simulink model "gm_iir_filter_simulink"  (R2025a)
settings: Solver=FixedStepAuto  StartTime=0.0  StopTime=5e-3  MaxStep=1/(44e3)  RelTol=1e-3  EnableMultiTasking=on
libraries: hdlmdlgenlib x17
settings Model: Creator=thiag  LastModifiedBy=thiag
settings SolverCC: PositivePriorityOrder=on
settings OptimizationCC: BlockReduction=off  ConditionallyExecuteInputs=off  DefaultParameterBehavior=Inlined  EnhancedBackFolding=on  PassReuseOutputArgsAs=Individual arguments  ZeroExternalMemoryAtStartup=off  ZeroInternalMemoryAtStartup=off  MaxStackSize=64  OptimizeBlockOrder=speed  DifferentSizesBufferReuse=on  OptimizationCustomize=off  EfficientTunableParamExpr=on
settings DebuggingCC: InheritedTsInSrcMsg=none  ParameterTunabilityLossMsg=error
settings HardwareCC: ProdBitPerPointer=32.0  ProdBitPerSizeT=32.0  ProdBitPerPtrDiffT=32.0  ProdLargestAtomicInteger=Long  ProdLargestAtomicFloat=Double  ProdWordSize=32.0  ProdLongLongMode=on  ProdHWDeviceType=ARM Compatible->ARM Cortex-A (32-bit)  TargetBitPerPointer=64.0  TargetBitPerSizeT=64.0  TargetBitPerPtrDiffT=64.0  TargetLongLongMode=on  TargetIntDivRoundTo=Zero  TargetEndianess=LittleEndian  TargetWordSize=64.0  TargetHWDeviceType=Custom Processor->MATLAB Host Computer  ProdEqTarget=off
settings RTWCC: SystemTargetFile=ert.tlc  HardwareBoard=Altera Cyclone V SoC development kit  TLCOptions="-aInlineSetEventsForThisBaseRateFcn=TLC_FALSE -aSuppressMultiTaskScheduler=TLC_FALSE  -aRateBasedStepFcn=0"  TemplateMakefile=ert_default_tmf  Toolchain=ARM Development Studio Altera Edition (DS-5 AE)  Description=Embedded Coder
settings CodeAppCC: ForceParamTrailComments=on  IgnoreCustomStorageClasses=off  OperatorAnnotations=on  SimulinkDataObjDesc=on  SFDataObjDesc=on  InsertBlockDesc=on
settings ERTTargetCC: ExtModeTransport=0.0  ExtModeStaticAlloc=off  ExtModeMexFile=ext_comm  ExtModeIntrfLevel=Level1

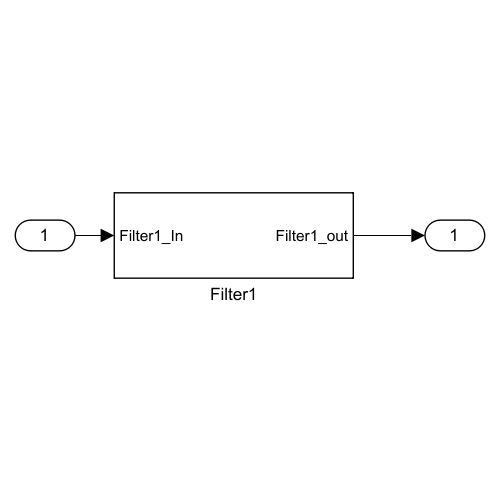
[thumbnail: Simulink's stored preview of the top-level diagram]
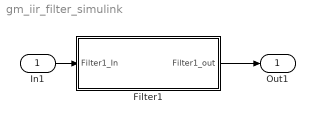
== system gm_iir_filter_simulink ==
  In1 : Inport  OutDataTypeStr=double  PortDimensions=1  SampleTime=0.0001
  Filter1 : Subsystem
  Out1 : Outport  SampleTime=0.0001  VectorParamsAs1DForOutWhenUnconnected=off
  wires:
  In1/1 -> Filter1/1(Filter1_In)
  Filter1/1(Filter1_out) -> Out1/1

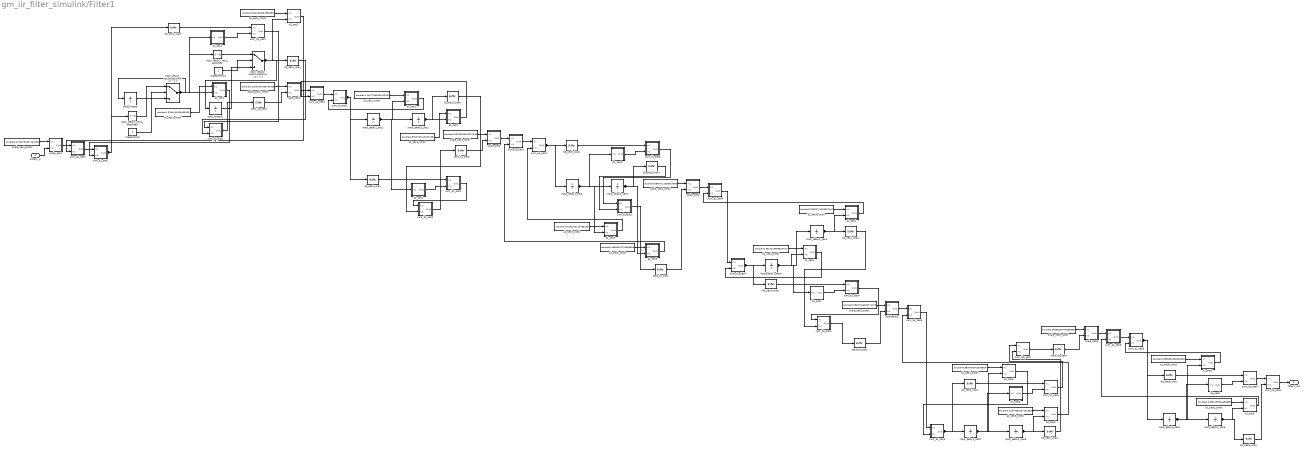
== system gm_iir_filter_simulink/Filter1 ==
  Filter1_In : Inport  OutDataTypeStr=double  SampleTime=0.0001
  a1_sec1 : Subsystem
      mask Display: disp('NFP\nmul');
  a1_sec1_const : Constant  Value=double(-1.3234411929489132)  OutDataTypeStr=double  SampleTime=0.0001
  a1_sec2 : Subsystem
      mask Display: disp('NFP\nmul');
  a1_sec2_const : Constant  Value=double(-1.1407793295142226)  OutDataTypeStr=double  SampleTime=0.0001
  a1_sec3 : Subsystem
      mask Display: disp('NFP\nmul');
  a1_sec3_const : Constant  Value=double(-1.0151579111465192)  OutDataTypeStr=double  SampleTime=0.0001
  a1_sec4 : Subsystem
      mask Display: disp('NFP\nmul');
  a1_sec4_const : Constant  Value=double(-0.9314129488925742)  OutDataTypeStr=double  SampleTime=0.0001
  a1_sec5 : Subsystem
      mask Display: disp('NFP\nmul');
  a1_sec5_const : Constant  Value=double(-0.8800759761000565)  OutDataTypeStr=double  SampleTime=0.0001
  a1_sec6 : Subsystem
      mask Display: disp('NFP\nmul');
  a1_sec6_const : Constant  Value=double(-0.8556632056226252)  OutDataTypeStr=double  SampleTime=0.0001
  a2_sec1 : Subsystem
      mask Display: disp('NFP\nmul');
  a2_sec1_const : Constant  Value=double(0.8342313264356033)  OutDataTypeStr=double  SampleTime=0.0001
  a2_sec2 : Subsystem
      mask Display: disp('NFP\nmul');
  a2_sec2_const : Constant  Value=double(0.5810700119457158)  OutDataTypeStr=double  SampleTime=0.0001
  a2_sec3 : Subsystem
      mask Display: disp('NFP\nmul');
  a2_sec3_const : Constant  Value=double(0.40696424731563696)  OutDataTypeStr=double  SampleTime=0.0001
  a2_sec4 : Subsystem
      mask Display: disp('NFP\nmul');
  a2_sec4_const : Constant  Value=double(0.29089741033357047)  OutDataTypeStr=double  SampleTime=0.0001
  a2_sec5 : Subsystem
      mask Display: disp('NFP\nmul');
  a2_sec5_const : Constant  Value=double(0.21974662237102355)  OutDataTypeStr=double  SampleTime=0.0001
  a2_sec6 : Subsystem
      mask Display: disp('NFP\nmul');
  a2_sec6_const : Constant  Value=double(0.18591159546286895)  OutDataTypeStr=double  SampleTime=0.0001
  b0_sec1_unary : hdlmdlgenlib/Buffer
  b0_sec2_unary : hdlmdlgenlib/Buffer
  b0_sec3_unary : hdlmdlgenlib/Buffer
  b0_sec4_unary : hdlmdlgenlib/Buffer
  b0_sec5_unary : hdlmdlgenlib/Buffer
  b0_sec6_unary : hdlmdlgenlib/Buffer
  b1_sec1 : Subsystem
      mask Display: disp('NFP\ngain_pow2');
  b1_sec2 : Subsystem
      mask Display: disp('NFP\ngain_pow2');
  b1_sec3 : Subsystem
      mask Display: disp('NFP\ngain_pow2');
  b1_sec4 : Subsystem
      mask Display: disp('NFP\ngain_pow2');
  b1_sec5 : Subsystem
      mask Display: disp('NFP\ngain_pow2');
  b1_sec6 : Subsystem
      mask Display: disp('NFP\ngain_pow2');
  b2_sec1_unary : hdlmdlgenlib/Buffer
  b2_sec2_unary : hdlmdlgenlib/Buffer
  b2_sec3_unary : hdlmdlgenlib/Buffer
  b2_sec4_unary : hdlmdlgenlib/Buffer
  b2_sec5_unary : hdlmdlgenlib/Buffer
  b2_sec6_unary : hdlmdlgenlib/Buffer
  input_delay1_sec1_absorbed : Delay  DelayLength=0
  input_delay1_sec1bypassMux : Switch  Criteria=u2 ~= 0  Threshold=double(0)  OutDataTypeStr=double  SampleTime=0.0001  SaturateOnIntegerOverflow=off  InputSameDT=off
  input_delay1_sec{2..6} (5 alike) : UnitDelay  InitialCondition=double(0)  SampleTime=0.0001
  input_delay2_sec1_absorbed : Delay  DelayLength=0
  input_delay2_sec1bypassMux : Switch  Criteria=u2 ~= 0  Threshold=double(0)  OutDataTypeStr=double  SampleTime=0.0001  SaturateOnIntegerOverflow=off  InputSameDT=off
  input_delay2_sec{2..6} (5 alike) : UnitDelay  InitialCondition=double(0)  SampleTime=0.0001
  out0_bypass : UnitDelay  SampleTime=0.0001
  out0_bypass1 : UnitDelay  SampleTime=0.0001
  scale_sec1 : Subsystem
      mask Display: disp('NFP\nmul');
  scale_sec1_const : Constant  Value=double(0.12769753337167256)  OutDataTypeStr=double  SampleTime=0.0001
  scale_sec2 : Subsystem
      mask Display: disp('NFP\nmul');
  scale_sec2_const : Constant  Value=double(0.11007267060787335)  OutDataTypeStr=double  SampleTime=0.0001
  scale_sec3 : Subsystem
      mask Display: disp('NFP\nmul');
  scale_sec3_const : Constant  Value=double(0.09795158404227945)  OutDataTypeStr=double  SampleTime=0.0001
  scale_sec4 : Subsystem
      mask Display: disp('NFP\nmul');
  scale_sec4_const : Constant  Value=double(0.08987111536024908)  OutDataTypeStr=double  SampleTime=0.0001
  scale_sec5 : Subsystem
      mask Display: disp('NFP\nmul');
  scale_sec5_const : Constant  Value=double(0.08491766156774178)  OutDataTypeStr=double  SampleTime=0.0001
  scale_sec6 : Subsystem
      mask Display: disp('NFP\nmul');
  scale_sec6_const : Constant  Value=double(0.08256209746006095)  OutDataTypeStr=double  SampleTime=0.0001
  sec1_to_sec2 : hdlmdlgenlib/Buffer
  sec2_to_sec3 : hdlmdlgenlib/Buffer
  sec3_to_sec4 : hdlmdlgenlib/Buffer
  sec4_to_sec5 : hdlmdlgenlib/Buffer
  sec5_to_sec6 : hdlmdlgenlib/Buffer
  stateControl : Constant  OutDataTypeStr=boolean  SampleTime=0.0001
  stateControl1 : Constant  OutDataTypeStr=boolean  SampleTime=0.0001
  sum_a1_sec1 : Subsystem
      mask Display: disp('NFP\nadd');
  sum_a1_sec2 : Subsystem
      mask Display: disp('NFP\nadd');
  sum_a1_sec3 : Subsystem
      mask Display: disp('NFP\nadd');
  sum_a1_sec4 : Subsystem
      mask Display: disp('NFP\nadd');
  sum_a1_sec5 : Subsystem
      mask Display: disp('NFP\nadd');
  sum_a1_sec6 : Subsystem
      mask Display: disp('NFP\nadd');
  sum_a2_sec1 : Subsystem
      mask Display: disp('NFP\nadd');
  sum_a2_sec2 : Subsystem
      mask Display: disp('NFP\nadd');
  sum_a2_sec3 : Subsystem
      mask Display: disp('NFP\nadd');
  sum_a2_sec4 : Subsystem
      mask Display: disp('NFP\nadd');
  sum_a2_sec5 : Subsystem
      mask Display: disp('NFP\nadd');
  sum_a2_sec6 : Subsystem
      mask Display: disp('NFP\nadd');
  sum_b1_sec1 : Subsystem
      mask Display: disp('NFP\nadd');
  sum_b1_sec2 : Subsystem
      mask Display: disp('NFP\nadd');
  sum_b1_sec3 : Subsystem
      mask Display: disp('NFP\nadd');
  sum_b1_sec4 : Subsystem
      mask Display: disp('NFP\nadd');
  sum_b1_sec5 : Subsystem
      mask Display: disp('NFP\nadd');
  sum_b1_sec6 : Subsystem
      mask Display: disp('NFP\nadd');
  sum_b2_sec1 : Subsystem
      mask Display: disp('NFP\nadd');
  sum_b2_sec2 : Subsystem
      mask Display: disp('NFP\nadd');
  sum_b2_sec3 : Subsystem
      mask Display: disp('NFP\nadd');
  sum_b2_sec4 : Subsystem
      mask Display: disp('NFP\nadd');
  sum_b2_sec5 : Subsystem
      mask Display: disp('NFP\nadd');
  sum_b2_sec6 : Subsystem
      mask Display: disp('NFP\nadd');
  Filter1_out : Outport  OutDataTypeStr=double  SampleTime=0.0001
  wires:
  sec2_to_sec3/1 -> scale_sec3/2(In2)
  scale_sec1_const/1 -> scale_sec1/1(In1)
  input_delay2_sec4/1 -> b2_sec4_unary/1, a2_sec4/2(In2)
  sum_a1_sec2/1(Out1) -> b0_sec2_unary/1, input_delay1_sec2/1
  sum_a2_sec1/1(Out1) -> sum_a1_sec1/1(In1)
  Filter1_In/1 -> scale_sec1/2(In2)
  input_delay1_sec1_absorbed/1 -> input_delay1_sec1bypassMux/1
  sum_a1_sec1/1(Out1) -> b0_sec1_unary/1, input_delay1_sec1_absorbed/1
  scale_sec1/1(Out1) -> sum_a2_sec1/1(In1)
  out0_bypass/1 -> input_delay1_sec1bypassMux/3
  sum_b2_sec2/1(Out1) -> sec2_to_sec3/1
  stateControl/1 -> input_delay1_sec1bypassMux/2
  b0_sec1_unary/1 -> sum_b1_sec1/1(In1)
  input_delay1_sec1bypassMux/1 -> out0_bypass/1, input_delay2_sec1_absorbed/1, a1_sec1/2(In2), b1_sec1/1(In1)
  b0_sec4_unary/1 -> sum_b1_sec4/1(In1)
  b0_sec3_unary/1 -> sum_b1_sec3/1(In1)
  a1_sec1_const/1 -> a1_sec1/1(In1)
  a1_sec2/1(Out1) -> sum_a1_sec2/2(In2)
  b1_sec1/1(Out1) -> sum_b1_sec1/2(In2)
  sum_b1_sec2/1(Out1) -> sum_b2_sec2/1(In1)
  input_delay2_sec1_absorbed/1 -> input_delay2_sec1bypassMux/1
  scale_sec3/1(Out1) -> sum_a2_sec3/1(In1)
  input_delay2_sec2/1 -> b2_sec2_unary/1, a2_sec2/2(In2)
  b0_sec2_unary/1 -> sum_b1_sec2/1(In1)
  stateControl1/1 -> input_delay2_sec1bypassMux/2
  a2_sec2/1(Out1) -> sum_a2_sec2/2(In2)
  a1_sec1/1(Out1) -> sum_a1_sec1/2(In2)
  b1_sec5/1(Out1) -> sum_b1_sec5/2(In2)
  sec1_to_sec2/1 -> scale_sec2/2(In2)
  out0_bypass1/1 -> input_delay2_sec1bypassMux/3
  a2_sec1/1(Out1) -> sum_a2_sec1/2(In2)
  sum_b2_sec1/1(Out1) -> sec1_to_sec2/1
  a2_sec3/1(Out1) -> sum_a2_sec3/2(In2)
  input_delay2_sec1bypassMux/1 -> out0_bypass1/1, a2_sec1/2(In2), b2_sec1_unary/1
  b1_sec3/1(Out1) -> sum_b1_sec3/2(In2)
  scale_sec2/1(Out1) -> sum_a2_sec2/1(In1)
  a2_sec1_const/1 -> a2_sec1/1(In1)
  sum_b1_sec1/1(Out1) -> sum_b2_sec1/1(In1)
  scale_sec2_const/1 -> scale_sec2/1(In1)
  input_delay1_sec4/1 -> b1_sec4/1(In1), a1_sec4/2(In2), input_delay2_sec4/1
  b2_sec1_unary/1 -> sum_b2_sec1/2(In2)
  b2_sec2_unary/1 -> sum_b2_sec2/2(In2)
  sum_a2_sec2/1(Out1) -> sum_a1_sec2/1(In1)
  a1_sec2_const/1 -> a1_sec2/1(In1)
  scale_sec3_const/1 -> scale_sec3/1(In1)
  input_delay1_sec2/1 -> b1_sec2/1(In1), a1_sec2/2(In2), input_delay2_sec2/1
  a2_sec2_const/1 -> a2_sec2/1(In1)
  b1_sec2/1(Out1) -> sum_b1_sec2/2(In2)
  sum_a2_sec3/1(Out1) -> sum_a1_sec3/1(In1)
  sum_a1_sec3/1(Out1) -> input_delay1_sec3/1, b0_sec3_unary/1
  sec3_to_sec4/1 -> scale_sec4/2(In2)
  b2_sec3_unary/1 -> sum_b2_sec3/2(In2)
  b2_sec5_unary/1 -> sum_b2_sec5/2(In2)
  input_delay1_sec3/1 -> b1_sec3/1(In1), a1_sec3/2(In2), input_delay2_sec3/1
  input_delay2_sec3/1 -> b2_sec3_unary/1, a2_sec3/2(In2)
  a1_sec3_const/1 -> a1_sec3/1(In1)
  sum_b2_sec3/1(Out1) -> sec3_to_sec4/1
  scale_sec4/1(Out1) -> sum_a2_sec4/1(In1)
  a1_sec3/1(Out1) -> sum_a1_sec3/2(In2)
  a2_sec3_const/1 -> a2_sec3/1(In1)
  sum_b1_sec3/1(Out1) -> sum_b2_sec3/1(In1)
  scale_sec4_const/1 -> scale_sec4/1(In1)
  sum_a2_sec4/1(Out1) -> sum_a1_sec4/1(In1)
  sum_a1_sec4/1(Out1) -> b0_sec4_unary/1, input_delay1_sec4/1
  a1_sec4_const/1 -> a1_sec4/1(In1)
  a2_sec4_const/1 -> a2_sec4/1(In1)
  a1_sec4/1(Out1) -> sum_a1_sec4/2(In2)
  b1_sec4/1(Out1) -> sum_b1_sec4/2(In2)
  sum_b2_sec4/1(Out1) -> sec4_to_sec5/1
  a2_sec4/1(Out1) -> sum_a2_sec4/2(In2)
  b2_sec4_unary/1 -> sum_b2_sec4/2(In2)
  sum_b1_sec4/1(Out1) -> sum_b2_sec4/1(In1)
  scale_sec5_const/1 -> scale_sec5/1(In1)
  sec4_to_sec5/1 -> scale_sec5/2(In2)
  scale_sec5/1(Out1) -> sum_a2_sec5/1(In1)
  sum_a2_sec5/1(Out1) -> sum_a1_sec5/1(In1)
  sum_a1_sec5/1(Out1) -> b0_sec5_unary/1, input_delay1_sec5/1
  a1_sec5_const/1 -> a1_sec5/1(In1)
  b0_sec5_unary/1 -> sum_b1_sec5/1(In1)
  sum_a1_sec6/1(Out1) -> b0_sec6_unary/1, input_delay1_sec6/1
  input_delay1_sec5/1 -> b1_sec5/1(In1), a1_sec5/2(In2), input_delay2_sec5/1
  sum_b2_sec5/1(Out1) -> sec5_to_sec6/1
  a1_sec5/1(Out1) -> sum_a1_sec5/2(In2)
  a2_sec5_const/1 -> a2_sec5/1(In1)
  input_delay2_sec5/1 -> b2_sec5_unary/1, a2_sec5/2(In2)
  scale_sec6_const/1 -> scale_sec6/1(In1)
  sec5_to_sec6/1 -> scale_sec6/2(In2)
  sum_b1_sec5/1(Out1) -> sum_b2_sec5/1(In1)
  a2_sec5/1(Out1) -> sum_a2_sec5/2(In2)
  scale_sec6/1(Out1) -> sum_a2_sec6/1(In1)
  sum_a2_sec6/1(Out1) -> sum_a1_sec6/1(In1)
  a1_sec6_const/1 -> a1_sec6/1(In1)
  b0_sec6_unary/1 -> sum_b1_sec6/1(In1)
  input_delay1_sec6/1 -> b1_sec6/1(In1), a1_sec6/2(In2), input_delay2_sec6/1
  a1_sec6/1(Out1) -> sum_a1_sec6/2(In2)
  b2_sec6_unary/1 -> sum_b2_sec6/2(In2)
  b1_sec6/1(Out1) -> sum_b1_sec6/2(In2)
  a2_sec6_const/1 -> a2_sec6/1(In1)
  input_delay2_sec6/1 -> a2_sec6/2(In2), b2_sec6_unary/1
  sum_b1_sec6/1(Out1) -> sum_b2_sec6/1(In1)
  a2_sec6/1(Out1) -> sum_a2_sec6/2(In2)
  sum_b2_sec6/1(Out1) -> Filter1_out/1

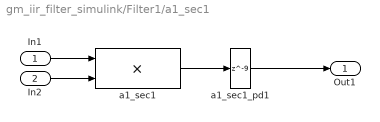
== system gm_iir_filter_simulink/Filter1/a1_sec1 ==
  In1 : Inport
  In2 : Inport  Port=2
  a1_sec1 : Product  Inputs=**  OutDataTypeStr=double  SampleTime=0.0001
  a1_sec1_pd1 : Delay  DelayLength=9
  Out1 : Outport
  wires:
  In1/1 -> a1_sec1/1
  In2/1 -> a1_sec1/2
  a1_sec1/1 -> a1_sec1_pd1/1
  a1_sec1_pd1/1 -> Out1/1

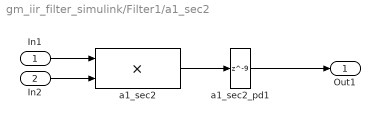
== system gm_iir_filter_simulink/Filter1/a1_sec2 ==
  In1 : Inport
  In2 : Inport  Port=2
  a1_sec2 : Product  Inputs=**  OutDataTypeStr=double  SampleTime=0.0001
  a1_sec2_pd1 : Delay  DelayLength=9
  Out1 : Outport
  wires:
  In1/1 -> a1_sec2/1
  In2/1 -> a1_sec2/2
  a1_sec2/1 -> a1_sec2_pd1/1
  a1_sec2_pd1/1 -> Out1/1

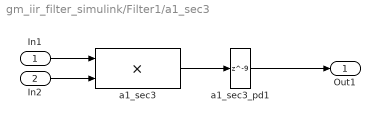
== system gm_iir_filter_simulink/Filter1/a1_sec3 ==
  In1 : Inport
  In2 : Inport  Port=2
  a1_sec3 : Product  Inputs=**  OutDataTypeStr=double  SampleTime=0.0001
  a1_sec3_pd1 : Delay  DelayLength=9
  Out1 : Outport
  wires:
  In1/1 -> a1_sec3/1
  In2/1 -> a1_sec3/2
  a1_sec3/1 -> a1_sec3_pd1/1
  a1_sec3_pd1/1 -> Out1/1

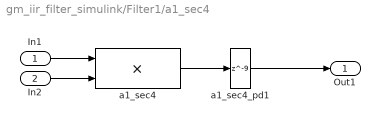
== system gm_iir_filter_simulink/Filter1/a1_sec4 ==
  In1 : Inport
  In2 : Inport  Port=2
  a1_sec4 : Product  Inputs=**  OutDataTypeStr=double  SampleTime=0.0001
  a1_sec4_pd1 : Delay  DelayLength=9
  Out1 : Outport
  wires:
  In1/1 -> a1_sec4/1
  In2/1 -> a1_sec4/2
  a1_sec4/1 -> a1_sec4_pd1/1
  a1_sec4_pd1/1 -> Out1/1

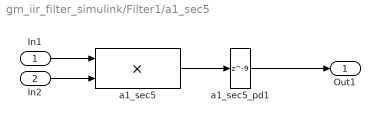
== system gm_iir_filter_simulink/Filter1/a1_sec5 ==
  In1 : Inport
  In2 : Inport  Port=2
  a1_sec5 : Product  Inputs=**  OutDataTypeStr=double  SampleTime=0.0001
  a1_sec5_pd1 : Delay  DelayLength=9
  Out1 : Outport
  wires:
  In1/1 -> a1_sec5/1
  In2/1 -> a1_sec5/2
  a1_sec5/1 -> a1_sec5_pd1/1
  a1_sec5_pd1/1 -> Out1/1

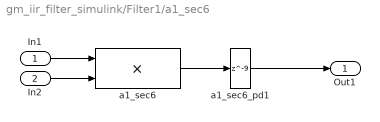
== system gm_iir_filter_simulink/Filter1/a1_sec6 ==
  In1 : Inport
  In2 : Inport  Port=2
  a1_sec6 : Product  Inputs=**  OutDataTypeStr=double  SampleTime=0.0001
  a1_sec6_pd1 : Delay  DelayLength=9
  Out1 : Outport
  wires:
  In1/1 -> a1_sec6/1
  In2/1 -> a1_sec6/2
  a1_sec6/1 -> a1_sec6_pd1/1
  a1_sec6_pd1/1 -> Out1/1

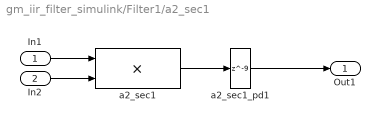
== system gm_iir_filter_simulink/Filter1/a2_sec1 ==
  In1 : Inport
  In2 : Inport  Port=2
  a2_sec1 : Product  Inputs=**  OutDataTypeStr=double  SampleTime=0.0001
  a2_sec1_pd1 : Delay  DelayLength=9
  Out1 : Outport
  wires:
  In1/1 -> a2_sec1/1
  In2/1 -> a2_sec1/2
  a2_sec1/1 -> a2_sec1_pd1/1
  a2_sec1_pd1/1 -> Out1/1

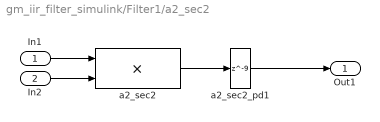
== system gm_iir_filter_simulink/Filter1/a2_sec2 ==
  In1 : Inport
  In2 : Inport  Port=2
  a2_sec2 : Product  Inputs=**  OutDataTypeStr=double  SampleTime=0.0001
  a2_sec2_pd1 : Delay  DelayLength=9
  Out1 : Outport
  wires:
  In1/1 -> a2_sec2/1
  In2/1 -> a2_sec2/2
  a2_sec2/1 -> a2_sec2_pd1/1
  a2_sec2_pd1/1 -> Out1/1

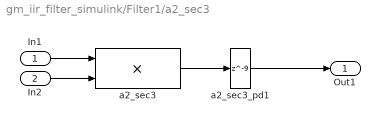
== system gm_iir_filter_simulink/Filter1/a2_sec3 ==
  In1 : Inport
  In2 : Inport  Port=2
  a2_sec3 : Product  Inputs=**  OutDataTypeStr=double  SampleTime=0.0001
  a2_sec3_pd1 : Delay  DelayLength=9
  Out1 : Outport
  wires:
  In1/1 -> a2_sec3/1
  In2/1 -> a2_sec3/2
  a2_sec3/1 -> a2_sec3_pd1/1
  a2_sec3_pd1/1 -> Out1/1

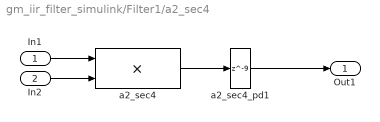
== system gm_iir_filter_simulink/Filter1/a2_sec4 ==
  In1 : Inport
  In2 : Inport  Port=2
  a2_sec4 : Product  Inputs=**  OutDataTypeStr=double  SampleTime=0.0001
  a2_sec4_pd1 : Delay  DelayLength=9
  Out1 : Outport
  wires:
  In1/1 -> a2_sec4/1
  In2/1 -> a2_sec4/2
  a2_sec4/1 -> a2_sec4_pd1/1
  a2_sec4_pd1/1 -> Out1/1

== system gm_iir_filter_simulink/Filter1/a2_sec5 ==
  In1 : Inport
  In2 : Inport  Port=2
  a2_sec5 : Product  Inputs=**  OutDataTypeStr=double  SampleTime=0.0001
  a2_sec5_pd1 : Delay  DelayLength=9
  Out1 : Outport
  wires:
  In1/1 -> a2_sec5/1
  In2/1 -> a2_sec5/2
  a2_sec5/1 -> a2_sec5_pd1/1
  a2_sec5_pd1/1 -> Out1/1

== system gm_iir_filter_simulink/Filter1/a2_sec6 ==
  In1 : Inport
  In2 : Inport  Port=2
  a2_sec6 : Product  Inputs=**  OutDataTypeStr=double  SampleTime=0.0001
  a2_sec6_pd1 : Delay  DelayLength=9
  Out1 : Outport
  wires:
  In1/1 -> a2_sec6/1
  In2/1 -> a2_sec6/2
  a2_sec6/1 -> a2_sec6_pd1/1
  a2_sec6_pd1/1 -> Out1/1

== system gm_iir_filter_simulink/Filter1/b1_sec1 ==
  In1 : Inport
  b1_sec1 : Gain  Gain=double(2)
  b1_sec1_pd1 : Delay
  Out1 : Outport
  wires:
  In1/1 -> b1_sec1/1
  b1_sec1/1 -> b1_sec1_pd1/1
  b1_sec1_pd1/1 -> Out1/1

== system gm_iir_filter_simulink/Filter1/b1_sec2 ==
  In1 : Inport
  b1_sec2 : Gain  Gain=double(2)
  b1_sec2_pd1 : Delay
  Out1 : Outport
  wires:
  In1/1 -> b1_sec2/1
  b1_sec2/1 -> b1_sec2_pd1/1
  b1_sec2_pd1/1 -> Out1/1

== system gm_iir_filter_simulink/Filter1/b1_sec3 ==
  In1 : Inport
  b1_sec3 : Gain  Gain=double(2)
  b1_sec3_pd1 : Delay
  Out1 : Outport
  wires:
  In1/1 -> b1_sec3/1
  b1_sec3/1 -> b1_sec3_pd1/1
  b1_sec3_pd1/1 -> Out1/1

== system gm_iir_filter_simulink/Filter1/b1_sec4 ==
  In1 : Inport
  b1_sec4 : Gain  Gain=double(2)
  b1_sec4_pd1 : Delay
  Out1 : Outport
  wires:
  In1/1 -> b1_sec4/1
  b1_sec4/1 -> b1_sec4_pd1/1
  b1_sec4_pd1/1 -> Out1/1

== system gm_iir_filter_simulink/Filter1/b1_sec5 ==
  In1 : Inport
  b1_sec5 : Gain  Gain=double(2)
  b1_sec5_pd1 : Delay
  Out1 : Outport
  wires:
  In1/1 -> b1_sec5/1
  b1_sec5/1 -> b1_sec5_pd1/1
  b1_sec5_pd1/1 -> Out1/1

== system gm_iir_filter_simulink/Filter1/b1_sec6 ==
  In1 : Inport
  b1_sec6 : Gain  Gain=double(2)
  b1_sec6_pd1 : Delay
  Out1 : Outport
  wires:
  In1/1 -> b1_sec6/1
  b1_sec6/1 -> b1_sec6_pd1/1
  b1_sec6_pd1/1 -> Out1/1

== system gm_iir_filter_simulink/Filter1/scale_sec1 ==
  In1 : Inport
  In2 : Inport  Port=2
  scale_sec1 : Product  Inputs=**  OutDataTypeStr=double  SampleTime=0.0001
  scale_sec1_pd1 : Delay  DelayLength=9
  Out1 : Outport
  wires:
  In1/1 -> scale_sec1/1
  In2/1 -> scale_sec1/2
  scale_sec1/1 -> scale_sec1_pd1/1
  scale_sec1_pd1/1 -> Out1/1

== system gm_iir_filter_simulink/Filter1/scale_sec2 ==
  In1 : Inport
  In2 : Inport  Port=2
  scale_sec2 : Product  Inputs=**  OutDataTypeStr=double  SampleTime=0.0001
  scale_sec2_pd1 : Delay  DelayLength=9
  Out1 : Outport
  wires:
  In1/1 -> scale_sec2/1
  In2/1 -> scale_sec2/2
  scale_sec2/1 -> scale_sec2_pd1/1
  scale_sec2_pd1/1 -> Out1/1

== system gm_iir_filter_simulink/Filter1/scale_sec3 ==
  In1 : Inport
  In2 : Inport  Port=2
  scale_sec3 : Product  Inputs=**  OutDataTypeStr=double  SampleTime=0.0001
  scale_sec3_pd1 : Delay  DelayLength=9
  Out1 : Outport
  wires:
  In1/1 -> scale_sec3/1
  In2/1 -> scale_sec3/2
  scale_sec3/1 -> scale_sec3_pd1/1
  scale_sec3_pd1/1 -> Out1/1

== system gm_iir_filter_simulink/Filter1/scale_sec4 ==
  In1 : Inport
  In2 : Inport  Port=2
  scale_sec4 : Product  Inputs=**  OutDataTypeStr=double  SampleTime=0.0001
  scale_sec4_pd1 : Delay  DelayLength=9
  Out1 : Outport
  wires:
  In1/1 -> scale_sec4/1
  In2/1 -> scale_sec4/2
  scale_sec4/1 -> scale_sec4_pd1/1
  scale_sec4_pd1/1 -> Out1/1

== system gm_iir_filter_simulink/Filter1/scale_sec5 ==
  In1 : Inport
  In2 : Inport  Port=2
  scale_sec5 : Product  Inputs=**  OutDataTypeStr=double  SampleTime=0.0001
  scale_sec5_pd1 : Delay  DelayLength=9
  Out1 : Outport
  wires:
  In1/1 -> scale_sec5/1
  In2/1 -> scale_sec5/2
  scale_sec5/1 -> scale_sec5_pd1/1
  scale_sec5_pd1/1 -> Out1/1

== system gm_iir_filter_simulink/Filter1/scale_sec6 ==
  In1 : Inport
  In2 : Inport  Port=2
  scale_sec6 : Product  Inputs=**  OutDataTypeStr=double  SampleTime=0.0001
  scale_sec6_pd1 : Delay  DelayLength=9
  Out1 : Outport
  wires:
  In1/1 -> scale_sec6/1
  In2/1 -> scale_sec6/2
  scale_sec6/1 -> scale_sec6_pd1/1
  scale_sec6_pd1/1 -> Out1/1

== system gm_iir_filter_simulink/Filter1/sum_a1_sec1 ==
  In1 : Inport
  In2 : Inport  Port=2
  sum_a1_sec1 : Sum  Inputs=+-  OutDataTypeStr=double  SampleTime=0.0001
  sum_a1_sec1_pd1 : Delay  DelayLength=11
  Out1 : Outport
  wires:
  In1/1 -> sum_a1_sec1/1
  In2/1 -> sum_a1_sec1/2
  sum_a1_sec1/1 -> sum_a1_sec1_pd1/1
  sum_a1_sec1_pd1/1 -> Out1/1

== system gm_iir_filter_simulink/Filter1/sum_a1_sec2 ==
  In1 : Inport
  In2 : Inport  Port=2
  sum_a1_sec2 : Sum  Inputs=+-  OutDataTypeStr=double  SampleTime=0.0001
  sum_a1_sec2_pd1 : Delay  DelayLength=11
  Out1 : Outport
  wires:
  In1/1 -> sum_a1_sec2/1
  In2/1 -> sum_a1_sec2/2
  sum_a1_sec2/1 -> sum_a1_sec2_pd1/1
  sum_a1_sec2_pd1/1 -> Out1/1

== system gm_iir_filter_simulink/Filter1/sum_a1_sec3 ==
  In1 : Inport
  In2 : Inport  Port=2
  sum_a1_sec3 : Sum  Inputs=+-  OutDataTypeStr=double  SampleTime=0.0001
  sum_a1_sec3_pd1 : Delay  DelayLength=11
  Out1 : Outport
  wires:
  In1/1 -> sum_a1_sec3/1
  In2/1 -> sum_a1_sec3/2
  sum_a1_sec3/1 -> sum_a1_sec3_pd1/1
  sum_a1_sec3_pd1/1 -> Out1/1

== system gm_iir_filter_simulink/Filter1/sum_a1_sec4 ==
  In1 : Inport
  In2 : Inport  Port=2
  sum_a1_sec4 : Sum  Inputs=+-  OutDataTypeStr=double  SampleTime=0.0001
  sum_a1_sec4_pd1 : Delay  DelayLength=11
  Out1 : Outport
  wires:
  In1/1 -> sum_a1_sec4/1
  In2/1 -> sum_a1_sec4/2
  sum_a1_sec4/1 -> sum_a1_sec4_pd1/1
  sum_a1_sec4_pd1/1 -> Out1/1

== system gm_iir_filter_simulink/Filter1/sum_a1_sec5 ==
  In1 : Inport
  In2 : Inport  Port=2
  sum_a1_sec5 : Sum  Inputs=+-  OutDataTypeStr=double  SampleTime=0.0001
  sum_a1_sec5_pd1 : Delay  DelayLength=11
  Out1 : Outport
  wires:
  In1/1 -> sum_a1_sec5/1
  In2/1 -> sum_a1_sec5/2
  sum_a1_sec5/1 -> sum_a1_sec5_pd1/1
  sum_a1_sec5_pd1/1 -> Out1/1

== system gm_iir_filter_simulink/Filter1/sum_a1_sec6 ==
  In1 : Inport
  In2 : Inport  Port=2
  sum_a1_sec6 : Sum  Inputs=+-  OutDataTypeStr=double  SampleTime=0.0001
  sum_a1_sec6_pd1 : Delay  DelayLength=11
  Out1 : Outport
  wires:
  In1/1 -> sum_a1_sec6/1
  In2/1 -> sum_a1_sec6/2
  sum_a1_sec6/1 -> sum_a1_sec6_pd1/1
  sum_a1_sec6_pd1/1 -> Out1/1

== system gm_iir_filter_simulink/Filter1/sum_a2_sec1 ==
  In1 : Inport
  In2 : Inport  Port=2
  sum_a2_sec1 : Sum  Inputs=+-  OutDataTypeStr=double  SampleTime=0.0001
  sum_a2_sec1_pd1 : Delay  DelayLength=11
  Out1 : Outport
  wires:
  In1/1 -> sum_a2_sec1/1
  In2/1 -> sum_a2_sec1/2
  sum_a2_sec1/1 -> sum_a2_sec1_pd1/1
  sum_a2_sec1_pd1/1 -> Out1/1

== system gm_iir_filter_simulink/Filter1/sum_a2_sec2 ==
  In1 : Inport
  In2 : Inport  Port=2
  sum_a2_sec2 : Sum  Inputs=+-  OutDataTypeStr=double  SampleTime=0.0001
  sum_a2_sec2_pd1 : Delay  DelayLength=11
  Out1 : Outport
  wires:
  In1/1 -> sum_a2_sec2/1
  In2/1 -> sum_a2_sec2/2
  sum_a2_sec2/1 -> sum_a2_sec2_pd1/1
  sum_a2_sec2_pd1/1 -> Out1/1

== system gm_iir_filter_simulink/Filter1/sum_a2_sec3 ==
  In1 : Inport
  In2 : Inport  Port=2
  sum_a2_sec3 : Sum  Inputs=+-  OutDataTypeStr=double  SampleTime=0.0001
  sum_a2_sec3_pd1 : Delay  DelayLength=11
  Out1 : Outport
  wires:
  In1/1 -> sum_a2_sec3/1
  In2/1 -> sum_a2_sec3/2
  sum_a2_sec3/1 -> sum_a2_sec3_pd1/1
  sum_a2_sec3_pd1/1 -> Out1/1

== system gm_iir_filter_simulink/Filter1/sum_a2_sec4 ==
  In1 : Inport
  In2 : Inport  Port=2
  sum_a2_sec4 : Sum  Inputs=+-  OutDataTypeStr=double  SampleTime=0.0001
  sum_a2_sec4_pd1 : Delay  DelayLength=11
  Out1 : Outport
  wires:
  In1/1 -> sum_a2_sec4/1
  In2/1 -> sum_a2_sec4/2
  sum_a2_sec4/1 -> sum_a2_sec4_pd1/1
  sum_a2_sec4_pd1/1 -> Out1/1

== system gm_iir_filter_simulink/Filter1/sum_a2_sec5 ==
  In1 : Inport
  In2 : Inport  Port=2
  sum_a2_sec5 : Sum  Inputs=+-  OutDataTypeStr=double  SampleTime=0.0001
  sum_a2_sec5_pd1 : Delay  DelayLength=11
  Out1 : Outport
  wires:
  In1/1 -> sum_a2_sec5/1
  In2/1 -> sum_a2_sec5/2
  sum_a2_sec5/1 -> sum_a2_sec5_pd1/1
  sum_a2_sec5_pd1/1 -> Out1/1

== system gm_iir_filter_simulink/Filter1/sum_a2_sec6 ==
  In1 : Inport
  In2 : Inport  Port=2
  sum_a2_sec6 : Sum  Inputs=+-  OutDataTypeStr=double  SampleTime=0.0001
  sum_a2_sec6_pd1 : Delay  DelayLength=11
  Out1 : Outport
  wires:
  In1/1 -> sum_a2_sec6/1
  In2/1 -> sum_a2_sec6/2
  sum_a2_sec6/1 -> sum_a2_sec6_pd1/1
  sum_a2_sec6_pd1/1 -> Out1/1

== system gm_iir_filter_simulink/Filter1/sum_b1_sec1 ==
  In1 : Inport
  In2 : Inport  Port=2
  sum_b1_sec1 : Sum  OutDataTypeStr=double  SampleTime=0.0001
  sum_b1_sec1_pd1 : Delay  DelayLength=11
  Out1 : Outport
  wires:
  In1/1 -> sum_b1_sec1/1
  In2/1 -> sum_b1_sec1/2
  sum_b1_sec1/1 -> sum_b1_sec1_pd1/1
  sum_b1_sec1_pd1/1 -> Out1/1

== system gm_iir_filter_simulink/Filter1/sum_b1_sec2 ==
  In1 : Inport
  In2 : Inport  Port=2
  sum_b1_sec2 : Sum  OutDataTypeStr=double  SampleTime=0.0001
  sum_b1_sec2_pd1 : Delay  DelayLength=11
  Out1 : Outport
  wires:
  In1/1 -> sum_b1_sec2/1
  In2/1 -> sum_b1_sec2/2
  sum_b1_sec2/1 -> sum_b1_sec2_pd1/1
  sum_b1_sec2_pd1/1 -> Out1/1

== system gm_iir_filter_simulink/Filter1/sum_b1_sec3 ==
  In1 : Inport
  In2 : Inport  Port=2
  sum_b1_sec3 : Sum  OutDataTypeStr=double  SampleTime=0.0001
  sum_b1_sec3_pd1 : Delay  DelayLength=11
  Out1 : Outport
  wires:
  In1/1 -> sum_b1_sec3/1
  In2/1 -> sum_b1_sec3/2
  sum_b1_sec3/1 -> sum_b1_sec3_pd1/1
  sum_b1_sec3_pd1/1 -> Out1/1

== system gm_iir_filter_simulink/Filter1/sum_b1_sec4 ==
  In1 : Inport
  In2 : Inport  Port=2
  sum_b1_sec4 : Sum  OutDataTypeStr=double  SampleTime=0.0001
  sum_b1_sec4_pd1 : Delay  DelayLength=11
  Out1 : Outport
  wires:
  In1/1 -> sum_b1_sec4/1
  In2/1 -> sum_b1_sec4/2
  sum_b1_sec4/1 -> sum_b1_sec4_pd1/1
  sum_b1_sec4_pd1/1 -> Out1/1

== system gm_iir_filter_simulink/Filter1/sum_b1_sec5 ==
  In1 : Inport
  In2 : Inport  Port=2
  sum_b1_sec5 : Sum  OutDataTypeStr=double  SampleTime=0.0001
  sum_b1_sec5_pd1 : Delay  DelayLength=11
  Out1 : Outport
  wires:
  In1/1 -> sum_b1_sec5/1
  In2/1 -> sum_b1_sec5/2
  sum_b1_sec5/1 -> sum_b1_sec5_pd1/1
  sum_b1_sec5_pd1/1 -> Out1/1

== system gm_iir_filter_simulink/Filter1/sum_b1_sec6 ==
  In1 : Inport
  In2 : Inport  Port=2
  sum_b1_sec6 : Sum  OutDataTypeStr=double  SampleTime=0.0001
  sum_b1_sec6_pd1 : Delay  DelayLength=11
  Out1 : Outport
  wires:
  In1/1 -> sum_b1_sec6/1
  In2/1 -> sum_b1_sec6/2
  sum_b1_sec6/1 -> sum_b1_sec6_pd1/1
  sum_b1_sec6_pd1/1 -> Out1/1

== system gm_iir_filter_simulink/Filter1/sum_b2_sec1 ==
  In1 : Inport
  In2 : Inport  Port=2
  sum_b2_sec1 : Sum  OutDataTypeStr=double  SampleTime=0.0001
  sum_b2_sec1_pd1 : Delay  DelayLength=11
  Out1 : Outport
  wires:
  In1/1 -> sum_b2_sec1/1
  In2/1 -> sum_b2_sec1/2
  sum_b2_sec1/1 -> sum_b2_sec1_pd1/1
  sum_b2_sec1_pd1/1 -> Out1/1

== system gm_iir_filter_simulink/Filter1/sum_b2_sec2 ==
  In1 : Inport
  In2 : Inport  Port=2
  sum_b2_sec2 : Sum  OutDataTypeStr=double  SampleTime=0.0001
  sum_b2_sec2_pd1 : Delay  DelayLength=11
  Out1 : Outport
  wires:
  In1/1 -> sum_b2_sec2/1
  In2/1 -> sum_b2_sec2/2
  sum_b2_sec2/1 -> sum_b2_sec2_pd1/1
  sum_b2_sec2_pd1/1 -> Out1/1

== system gm_iir_filter_simulink/Filter1/sum_b2_sec3 ==
  In1 : Inport
  In2 : Inport  Port=2
  sum_b2_sec3 : Sum  OutDataTypeStr=double  SampleTime=0.0001
  sum_b2_sec3_pd1 : Delay  DelayLength=11
  Out1 : Outport
  wires:
  In1/1 -> sum_b2_sec3/1
  In2/1 -> sum_b2_sec3/2
  sum_b2_sec3/1 -> sum_b2_sec3_pd1/1
  sum_b2_sec3_pd1/1 -> Out1/1

== system gm_iir_filter_simulink/Filter1/sum_b2_sec4 ==
  In1 : Inport
  In2 : Inport  Port=2
  sum_b2_sec4 : Sum  OutDataTypeStr=double  SampleTime=0.0001
  sum_b2_sec4_pd1 : Delay  DelayLength=11
  Out1 : Outport
  wires:
  In1/1 -> sum_b2_sec4/1
  In2/1 -> sum_b2_sec4/2
  sum_b2_sec4/1 -> sum_b2_sec4_pd1/1
  sum_b2_sec4_pd1/1 -> Out1/1

== system gm_iir_filter_simulink/Filter1/sum_b2_sec5 ==
  In1 : Inport
  In2 : Inport  Port=2
  sum_b2_sec5 : Sum  OutDataTypeStr=double  SampleTime=0.0001
  sum_b2_sec5_pd1 : Delay  DelayLength=11
  Out1 : Outport
  wires:
  In1/1 -> sum_b2_sec5/1
  In2/1 -> sum_b2_sec5/2
  sum_b2_sec5/1 -> sum_b2_sec5_pd1/1
  sum_b2_sec5_pd1/1 -> Out1/1

== system gm_iir_filter_simulink/Filter1/sum_b2_sec6 ==
  In1 : Inport
  In2 : Inport  Port=2
  sum_b2_sec6 : Sum  OutDataTypeStr=double  SampleTime=0.0001
  sum_b2_sec6_pd1 : Delay  DelayLength=11
  Out1 : Outport
  wires:
  In1/1 -> sum_b2_sec6/1
  In2/1 -> sum_b2_sec6/2
  sum_b2_sec6/1 -> sum_b2_sec6_pd1/1
  sum_b2_sec6_pd1/1 -> Out1/1
